simulink model "FloatingOffshoreWind_ForceRAO"  (R2020b)
settings: Solver=ode4  StartTime=0.0  StopTime=200  FixedStep=0.1  RelTol=1e-3  EnableMultiTasking=on
undefined symbols (not defined in the file): slcm, vessel, vesselABC
libraries: simulink_extras x6, mssSimulink x5, simulink x1
settings Model: Creator=Thor  LastModifiedBy=thor
settings DataIOCC: LimitDataPoints=on  SaveFormat=Array  SignalLoggingSaveFormat=ModelDataLogs  ReturnWorkspaceOutputs=off
settings OptimizationCC: ExpressionDepthLimit=2147483647  LifeSpan=inf
settings DebuggingCC: UnderspecifiedInitializationDetection=Classic  MergeDetectMultiDrivingBlocksExec=none  SolverPrmCheckMsg=warning  FcnCallInpInsideContextMsg=warning  StateNameClashWarn=warning  SFUnexpectedBacktrackingDiag=warning  SFNoUnconditionalDefaultTransitionDiag=warning  SFExecutionAtInitializationDiag=none  ArithmeticOperatorsInVariantConditions=warning
settings HardwareCC: ProdBitPerPointer=32  ProdBitPerSizeT=32  ProdBitPerPtrDiffT=32  ProdLargestAtomicFloat=None  ProdIntDivRoundTo=Undefined  ProdEndianess=Unspecified  ProdWordSize=32  ProdHWDeviceType=32-bit Generic
settings ModelReferenceCC: PropagateSignalLabelsOutOfModel=off
settings SFSimCC: SimUseLocalCustomCode=off  CustomCodeUndefinedFunction=UseInterfaceOnly
settings RTWCC: RTWUseLocalCustomCode=off
settings CodeAppCC: StateflowObjectComments=on
settings GRTTargetCC: TargetLangStandard=C89/C90 (ANSI)  CombineOutputUpdateFcns=off  GRTInterface=on
settings ConfigComp: CovMetricSettings=dw  CovSaveCumulativeToWorkspaceVar=on  CovSaveSingleToWorkspaceVar=on

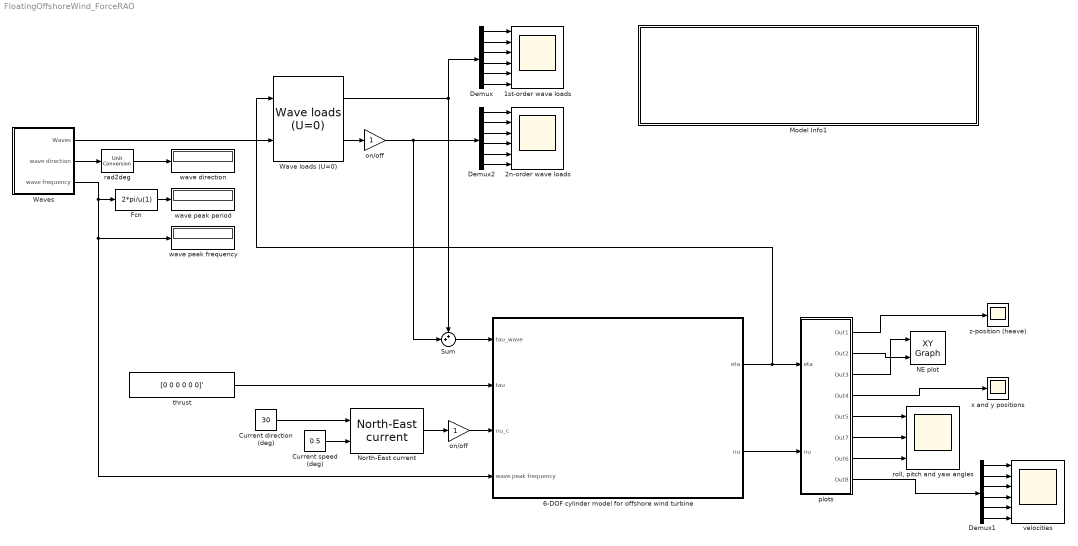
== system FloatingOffshoreWind_ForceRAO ==
  "1st-order wave loads " : Scope  NumInputPorts=6
  2n-order wave loads : Scope  NumInputPorts=6
  6-DOF cylinder model for offshore wind turbine : Subsystem  mask(6 DOF zero speed model){}
      mask help: System block containing the zero speed 6 DOF equations of motion.
      mask init:
      | load cylinder;
      | load cylinderABC;
      | ABC = vesselABC;
      mask Display: image('windturbine.jpg'); % Use "Edit Image" on toolstrip to change.
  Current direction (deg) : Constant  Value=30
  Current speed (deg) : Constant  Value=0.5
  Demux : Demux  Outputs=6
      settings: DisplayOption=none
  Demux1 : Demux  Outputs=6
      settings: DisplayOption=none
  Demux2 : Demux  Outputs=6
      settings: DisplayOption=none
  Fcn : Fcn  Expr=2*pi/u(1)
  Model Info1 : Subsystem  LoadFcn=slcm LoadBlock;  InitFcn=slcm('UpdateAllCMBlocksInThisModelInit')  mask(CMBlock){InitialSaveTempField=, InitialBlockCM=None, BlockCM=None, Frame=on, SaveTempField=, DisplayStringWithTags=|, MaskDisplayString=Offshore wind turbine modelled as a cylinder (D = 10.0 and T = 100.0 m) in WAMIT. \nThe wave-induced motions are computed using force RAOs. \n\nThe vessel simulator for stationkeeping in 6 DOFs is based on frequency-dependent hydrodynamic data. \nThe wave loads are computed using WAMIT data that are postprocessed by:\n\n>> vessel = wamit2vessel ('cylinder',100,10,10) generates the data structure 'vessel'\n\nThe data files are automatically loaded to the workspace before starting the simulation.\n\nAuthor: Thor I. Fossen\nTue Mar 09 08:00:28 2021, HorizontalTextAlignment=Left, LeftAlignmentValue=0.02, SourceBlockDiagram=DP_MotionRAO, TagMaxNumber=20, CMTag1=, CMTag2=, CMTag3=, CMTag4=, CMTag5=, CMTag6=, CMTag7=, CMTag8=, CMTag9=, CMTag10=, CMTag11=, CMTag12=, CMTag13=, CMTag14=, CMTag15=, CMTag16=, CMTag17=, CMTag18=, CMTag19=, CMTag20=}
      mask DisplayStringWithTags=|
      | Offshore wind turbine modelled as a cylinder (D = 10.0 and T = 100.0 m) in WAMIT.
      | The wave-induced motions are computed using force RAOs.
      |
      | The vessel simulator for stationkeeping in 6 DOFs is based on frequency-dependent hydrodynamic data.
      | The wave loads are computed using WAMIT data that are postprocessed by:
      |
      | >> vessel = wamit2vessel ('cylinder',100,10,10) generates the data structure 'vessel'
      |
      | The data files are automatically loaded to the workspace before starting the simulation.
      |
      | Author: Thor I. Fossen
      | %<LastModificationDate>
      mask help: This block allows revision control information to be displayed within the model.
      settings: CopyFcn=slcm CopyBlock;  DeleteFcn=slcm Cancel;  PostSaveFcn=slcm('UpdateAllCMBlocksInThisModel')  NameChangeFcn=slcm Rename;  OpenFcn=slcm
      mask Display: text(str2num(LeftAlignmentValue), 0.5, MaskDisplayString, 'HorizontalAlignment', HorizontalTextAlignment)
  NE plot : simulink/Sinks/XY Graph  xmin=-50  xmax=50  ymin=-50  ymax=50  st=-1
  "North-East current " : mssSimulink/Environment/Current/North-East current  SystemSampleTime=-1  VariantActivationTime=update diagram  Latency=0  AutoFrameSizeCalculation=off
  Sum : Sum  Inputs=++|
  "Wave loads (U=0) " : mssSimulink/Hydrodynamics/Wave loads (U=0)  SystemSampleTime=-1  VariantActivationTime=update diagram  Latency=0  AutoFrameSizeCalculation=off
  Waves : Subsystem  mask(Waves){spectrum_type=Jonswap, disp_flag=off, plot_spectrum=off, plot_realization=off, hs=5, omega_peak=2*pi/8, psi_mean=30*pi/180, gamma=3.3, spread=2, depth=inf, nfreq=20, ndir=10, energylim=0.005, freq_cutoff=3, dir_cutoff=0, rand_seed=0, rand_freq=on, rand_dir=on, Zeta_a=0, Omega=0, Phase=0, Wavenum=0, Psi=0}
      mask prompts: spectrum_type "Spectrum type"; disp_flag "Display initialization info in workspace window"; plot_spectrum "Plot spectrum"; plot_realization "Plot sea state realization (time-consuming)"; hs "Significant wave height Hs (m)"; omega_peak "Peak frequency omega_0 (rad/s)"; psi_mean "Mean wave direction (rad)"; gamma "Spectrum peakedness factor [1,7], 3.3 default, 0 for using DNV value"; spread "Wave spreading factor (1,2,3,4,5)"; depth "Average water depth (m), use inf for deep water"; nfreq "Number of frequencies in grid (recommended > 20)"; ndir "Number of directions in grid, 1 for long-crested waves"; energylim "Wave component energy limit [0 1] or number of waves (e.g. 50)"; freq_cutoff "Frequency cutoff factor [1.5, 5], default 3"; dir_cutoff "Direction cutoff [0, 3pi/8], default 0"; rand_seed "Random seed"; rand_freq "Random frequencies"; rand_dir "Random directions"; Zeta_a "Amplitude vector 'Zeta_a' (m)"; Omega "Frequency vector 'Omega' (rad/s)"; Phase "Phase vector 'Phase' (rad)"; Wavenum "Wavenumber vector 'Wavenum' (1/m)"; Psi "Direction vector 'Psi'  (rad)"
      mask help:
      | Calculate harmonic wave component parameters from a wave spectrum.
      | - Input one wave direction in the mask to get long-crested waves.
      | - Input zero peak frequency to get an expectation value from north sea statistical data.
      | - Input an integer > 1 for energylim to set the number of wave components fixed to nwaves = energylim.
      |
      | Copyright (C) 2004 NTNU
      | Author: Oyvind Notland Smogeli
      mask init:
      | if spectrum_type < 4
      | 	[Zeta_a, Omega, Phase, Wavenum, Psi] = Wave_init(spectrum_type, hs, omega_peak, psi_mean,...
      | 	gamma, spread, depth, nfreq, ndir, energylim, freq_cutoff, dir_cutoff, rand_freq, rand_dir,...
      | 	rand_seed, plot_spectrum, plot_realization, disp_flag);
      | end
      mask Help:
      | <font face="Arial">
      | <b>Project:</b> Marine Systems Simulator: MSS<br>
      | <br>
      | Define harmonic wave components describing the sea state by extracting
      | components from a given frequency and direction spectrum. The output from the
      | block is a bus containing the following wave parameter vectors:</font></p>
      | <p><font face="Arial"><b>Zeta_a</b>: Vector of harmonic wave amplitudes [m]<br>
      | <b>Omega: </b>Vector of harmonic wave frequencies [rad/s]<br>
      | <b>Phase: </b>Vector of harmonic wave phases (random) [rad]<br>
      | <b>Wavenum:</b> Vector of harmonic wave numbers [1/m]<br>
      | <b>Psi: </b>Vector of harmonic wave directions [rad]</font></p>
      | <p><font face="Arial">The time series of sea surface elevation Zeta(x,y,t) can
      | be obtained as</font></p>
      | <p><font face="Arial">Zeta(x,y,t) = Sum( Zeta_a(i)*cos(Omega(i)*t + Phase(i) - Wavenum(i)*(x*cos(Psi(i))
      | + y*sin(Psi(i)))) )</font></p>
      | <p><font face="Arial">where the sum is taken from i = 1 to i = n and n is the number of harmonic
      | wave components.</font></p>
      | <p>&nbsp;</p>
      | <p><font face="Arial">Input one wave direction to get long-crested waves.<br>
      | <br>
      | If the peak frequency is set to zero, then the peak frequency is obtained from
      | the sugnificant wave height usign a formula for the North Sea (Norsok):</font></p>
      | <p><font face="Arial">w0 = 2*pi/(4.883 + 2.68*Hs^0.54);</font></p>
      | 
      | <p>&nbsp;</p>
      | <p><font face="Arial">The energy limit (energylim) should be defined either as a positive factor
      | between 0 and 1, or as a positive integer. In the first case it will
      | discard all wave components with energy content less than this ratio of the
      | total energy content of the sea state. A recommended value is 0.005 or lower. In
      | the second case it will keep the nwaves = energylim most significant waves.</font></p>
      | <p>&nbsp;</p>
      | <p><font face="Arial">The wave elevation Zeta(x,y,t) at time t and at the coordinate (x,y) is found from the output vectors as:</font></p>
      | <p>&nbsp;</p>
      | <p><font face="Arial" color="#800000">References</font><ul>
      |   <li><font face="Arial">Sørensen, A.J. (2005) Lecture notes of TMR4240 &quot;Marine Cybernetics - Modelling and Control&quot;</font>
      |   <font face="Arial">Dept of Marine Technology NTNU.</font></li>
      |   <li><font face="Arial">Johannessen, K., T. S. Meling, S. Haver. Joint
      |   Distribution for Wind and<br>
      |   Waves in the Northern North Sea. IJOPE Vol. 12, No. 1, March 2002</font></li>
      |   <li>&nbsp;</li>
      |   </ul>
      | <p><font face="Arial">Johannessen, K., T. S. Meling, S. Haver. Joint
      | Distribution for Wind and<br>
      | Waves in the Northern North Sea. IJOPE Vol. 12, No. 1, March 2002</font><p>&nbsp;<p>
      |   <font face="Arial"><b>Author:</b> Øyvind Smogeli, September 2004 </font>
      | <p>&nbsp;</p>
      | <p>&nbsp;</p>
      mask TypeOptions spectrum_type: ITTC | Jonswap | Torsethaugen | Predefined waves
      mask Callback spectrum_type: Wave_callback;
  on/off : Gain
  "on/off " : Gain
  plots : Subsystem
      mask Display: disp('time-series')
  rad2deg : mssSimulink/Utilities/Math Operations/Unit Conversion  in=rad2deg
  "roll, pitch and yaw angles" : Scope  NumInputPorts=3
  thrust : Constant  Value=[0 0 0 0 0 0]'
  velocities : Scope  NumInputPorts=6
  wave direction : Display
  wave peak frequency : Display
  wave peak period : Display
  x and y positions : Scope
  z-position (heave) : Scope
  wires:
  plots/3(Out3) -> NE plot/1
  plots/2(Out2) -> NE plot/2
  plots/4(Out4) -> x and y positions/1
  plots/5(Out5) -> "roll, pitch and yaw angles"/1
  plots/6(Out7) -> "roll, pitch and yaw angles"/2
  plots/7(Out6) -> "roll, pitch and yaw angles"/3
  plots/1(Out1) -> z-position (heave)/1
  Demux1/1 -> velocities/1
  Demux1/2 -> velocities/2
  Demux1/3 -> velocities/3
  Demux1/4 -> velocities/4
  Demux1/5 -> velocities/5
  Demux1/6 -> velocities/6
  plots/8(Out8) -> Demux1/1
  6-DOF cylinder model for offshore wind turbine/1(eta) -> "Wave loads (U=0) "/1, plots/1(eta)
  6-DOF cylinder model for offshore wind turbine/2(nu) -> plots/2(nu)
  Demux/1 -> "1st-order wave loads "/1
  Demux/2 -> "1st-order wave loads "/2
  Demux/3 -> "1st-order wave loads "/3
  Demux/4 -> "1st-order wave loads "/4
  Demux/5 -> "1st-order wave loads "/5
  Demux/6 -> "1st-order wave loads "/6
  "Wave loads (U=0) "/2 -> on/off/1
  Waves/1(Waves) -> "Wave loads (U=0) "/2
  Waves/2(wave direction) -> rad2deg/1
  rad2deg/1 -> wave direction/1
  Demux2/1 -> 2n-order wave loads/1
  Demux2/2 -> 2n-order wave loads/2
  Demux2/3 -> 2n-order wave loads/3
  Demux2/4 -> 2n-order wave loads/4
  Demux2/5 -> 2n-order wave loads/5
  Demux2/6 -> 2n-order wave loads/6
  "Wave loads (U=0) "/1 -> Sum/1, Demux/1
  on/off/1 -> Demux2/1, Sum/2
  thrust/1 -> 6-DOF cylinder model for offshore wind turbine/2(tau)
  "North-East current "/1 -> "on/off "/1
  "on/off "/1 -> 6-DOF cylinder model for offshore wind turbine/3(nu_c)
  Current speed (deg)/1 -> "North-East current "/2
  Current direction (deg)/1 -> "North-East current "/1
  Sum/1 -> 6-DOF cylinder model for offshore wind turbine/1(tau_wave)
  Waves/3(wave frequency) -> Fcn/1, 6-DOF cylinder model for offshore wind turbine/4(wave peak frequency), wave peak frequency/1
  Fcn/1 -> wave peak period/1

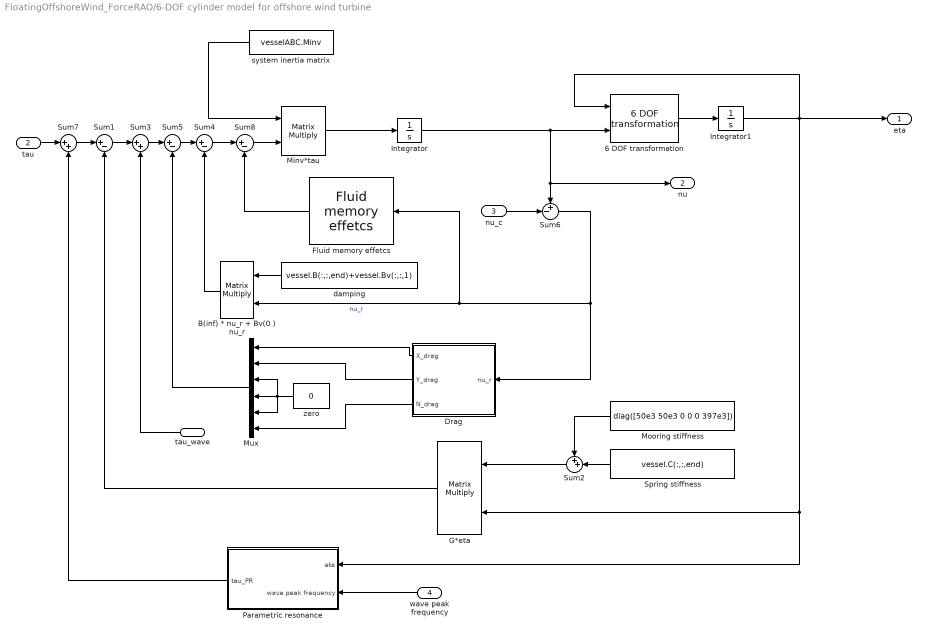
== system FloatingOffshoreWind_ForceRAO/6-DOF cylinder model for offshore wind turbine ==
  tau_wave : Inport
  tau : Inport  Port=2
  nu_c : Inport  Port=3
  wave peak frequency : Inport  Port=4
  "6 DOF transformation " : mssSimulink/Modelling/Kinematics/6 DOF transformation  SystemSampleTime=-1  VariantActivationTime=update diagram  Latency=0  AutoFrameSizeCalculation=off
  "B(inf) * nu_r + Bv(0 ) nu_r " : Product  Multiplication=Matrix(*)  SaturateOnIntegerOverflow=on  OutDataTypeStr=Inherit: Same as first input
  Drag : Subsystem  TreatAsAtomicUnit=on
  Fluid memory effetcs : mssSimulink/Hydrodynamics/Fluid memory effetcs  SystemSampleTime=-1  VariantActivationTime=update diagram  Latency=0  AutoFrameSizeCalculation=off
  G*eta : Product  Multiplication=Matrix(*)  SaturateOnIntegerOverflow=on  OutDataTypeStr=Inherit: Same as first input
  Integrator : Integrator  InitialCondition=[0.001 0.001 0.001 0.001 0.001 0.001]
  Integrator1 : Integrator
  Minv*tau : Product  Inputs=**  Multiplication=Matrix(*)  SaturateOnIntegerOverflow=on  OutDataTypeStr=Inherit: Same as first input
  Mooring stiffness : Constant  Value=diag([50e3 50e3 0 0 0 397e3])
  Mux : Mux  Inputs=6
  Parametric resonance : Subsystem
  Spring stiffness : Constant  Value=vessel.C(:,:,end)
  Sum{1,4..5,8} (4 alike) : Sum  Inputs=|+-  SaturateOnIntegerOverflow=on
  Sum2 : Sum  Inputs=++|  SaturateOnIntegerOverflow=on
  Sum3 : Sum  Inputs=|++  SaturateOnIntegerOverflow=on
  Sum6 : Sum  Inputs=+-|  SaturateOnIntegerOverflow=on
  Sum7 : Sum  Inputs=|++  SaturateOnIntegerOverflow=on
  damping : Constant  Value=vessel.B(:,:,end)+vessel.Bv(:,:,1)
  system inertia matrix : Constant  Value=vesselABC.Minv
  zero : Constant  Value=0
  eta : Outport
  nu : Outport  Port=2
  wires:
  "B(inf) * nu_r + Bv(0 ) nu_r "/1 -> Sum4/2
  Sum3/1 -> Sum5/1
  tau_wave/1 -> Sum3/2
  G*eta/1 -> Sum1/2
  Integrator1/1 -> eta/1, G*eta/2, Parametric resonance/1(eta), "6 DOF transformation "/1
  Spring stiffness/1 -> Sum2/2
  Sum1/1 -> Sum3/1
  Integrator/1 -> nu/1, Sum6/1, "6 DOF transformation "/2
  Drag/1(X_drag) -> Mux/1
  Drag/2(Y_drag) -> Mux/2
  Drag/3(N_drag) -> Mux/6
  zero/1 -> Mux/4, Mux/3, Mux/5
  Mux/1 -> Sum5/2
  Sum5/1 -> Sum4/1
  nu_c/1 -> Sum6/2
  Sum6/1 -> Fluid memory effetcs/1, "B(inf) * nu_r + Bv(0 ) nu_r "/2, Drag/1(nu_r)  "nu_r"
  tau/1 -> Sum7/1
  damping/1 -> "B(inf) * nu_r + Bv(0 ) nu_r "/1
  system inertia matrix/1 -> Minv*tau/1
  Minv*tau/1 -> Integrator/1
  "6 DOF transformation "/1 -> Integrator1/1
  Mooring stiffness/1 -> Sum2/1
  Sum2/1 -> G*eta/1
  Parametric resonance/1(tau_PR) -> Sum7/2
  Sum7/1 -> Sum1/1
  wave peak frequency/1 -> Parametric resonance/2(wave peak frequency)
  Sum4/1 -> Sum8/1
  Sum8/1 -> Minv*tau/2
  Fluid memory effetcs/1 -> Sum8/2

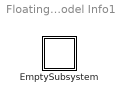
== system FloatingOffshoreWind_ForceRAO/Model Info1 ==
  EmptySubsystem : Subsystem

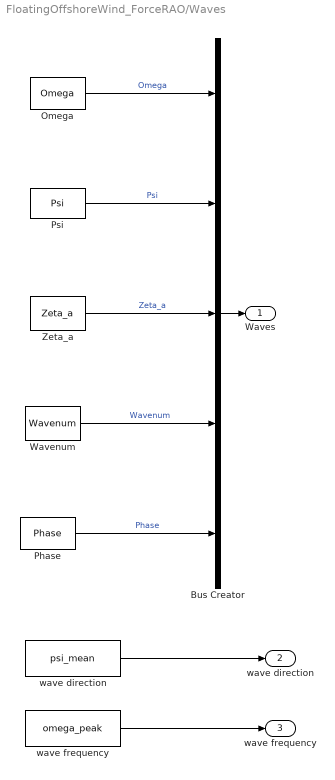
== system FloatingOffshoreWind_ForceRAO/Waves ==
  Bus Creator : BusCreator  Inputs=5
  Omega : Constant  Value=Omega
  Phase : Constant  Value=Phase
  Psi : Constant  Value=Psi
  Wavenum : Constant  Value=Wavenum
  Zeta_a : Constant  Value=Zeta_a
  "wave direction " : Constant  Value=psi_mean
  "wave frequency  " : Constant  Value=omega_peak
  Waves : Outport
  wave direction : Outport  Port=2
  wave frequency : Outport  Port=3
  wires:
  "wave direction "/1 -> wave direction/1
  Wavenum/1 -> Bus Creator/4  "Wavenum"
  Zeta_a/1 -> Bus Creator/3  "Zeta_a"
  Bus Creator/1 -> Waves/1
  Omega/1 -> Bus Creator/1  "Omega"
  Psi/1 -> Bus Creator/2  "Psi"
  Phase/1 -> Bus Creator/5  "Phase"
  "wave frequency  "/1 -> wave frequency/1

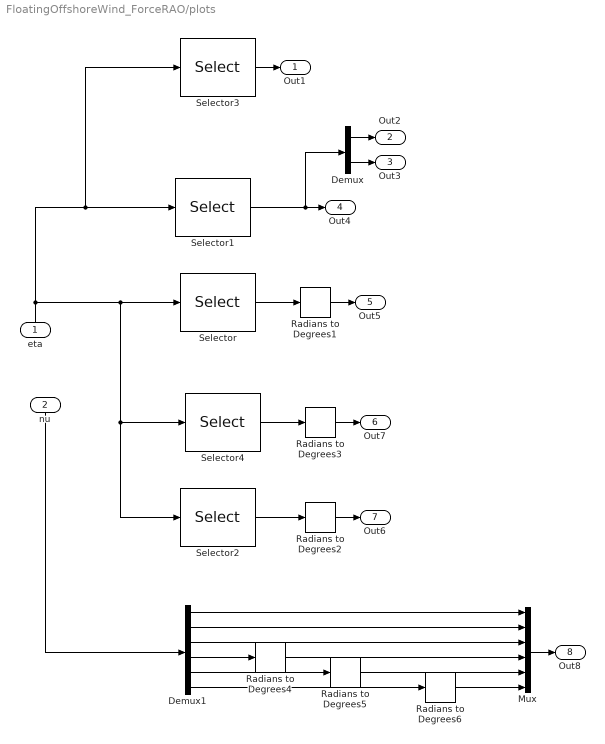
== system FloatingOffshoreWind_ForceRAO/plots ==
  eta : Inport
  nu : Inport  Port=2
  Demux : Demux  Outputs=2
      settings: DisplayOption=none
  Demux1 : Demux  Outputs=6
      settings: DisplayOption=none
  Mux : Mux  Inputs=6
  Radians to Degrees{1..6} (6 alike) : simulink_extras/Transformations/Radians to Degrees
  Selector : Selector  InputPortWidth=6  IndexOptions=Index vector (dialog)  Indices=[4 ]  OutputSizes=1
  Selector1 : Selector  InputPortWidth=6  IndexOptions=Index vector (dialog)  Indices=[1 2]  OutputSizes=1
  Selector2 : Selector  InputPortWidth=6  IndexOptions=Index vector (dialog)  Indices=[6]  OutputSizes=1
  Selector3 : Selector  InputPortWidth=6  IndexOptions=Index vector (dialog)  Indices=[3]  OutputSizes=1
  Selector4 : Selector  InputPortWidth=6  IndexOptions=Index vector (dialog)  Indices=[5]  OutputSizes=1
  Out1 : Outport
  Out2 : Outport  Port=2
  Out3 : Outport  Port=3
  Out4 : Outport  Port=4
  Out5 : Outport  Port=5
  Out7 : Outport  Port=6
  Out6 : Outport  Port=7
  Out8 : Outport  Port=8
  wires:
  eta/1 -> Selector3/1, Selector1/1, Selector/1, Selector2/1, Selector4/1
  Selector/1 -> Radians to Degrees1/1
  Selector1/1 -> Demux/1, Out4/1
  Selector2/1 -> Radians to Degrees2/1
  Selector3/1 -> Out1/1
  Demux/1 -> Out2/1
  Demux/2 -> Out3/1
  Radians to Degrees1/1 -> Out5/1
  Radians to Degrees2/1 -> Out6/1
  Selector4/1 -> Radians to Degrees3/1
  Radians to Degrees3/1 -> Out7/1
  nu/1 -> Demux1/1
  Demux1/1 -> Mux/1
  Demux1/2 -> Mux/2
  Demux1/3 -> Mux/3
  Demux1/4 -> Radians to Degrees4/1
  Demux1/5 -> Radians to Degrees5/1
  Demux1/6 -> Radians to Degrees6/1
  Radians to Degrees6/1 -> Mux/6
  Radians to Degrees5/1 -> Mux/5
  Radians to Degrees4/1 -> Mux/4
  Mux/1 -> Out8/1

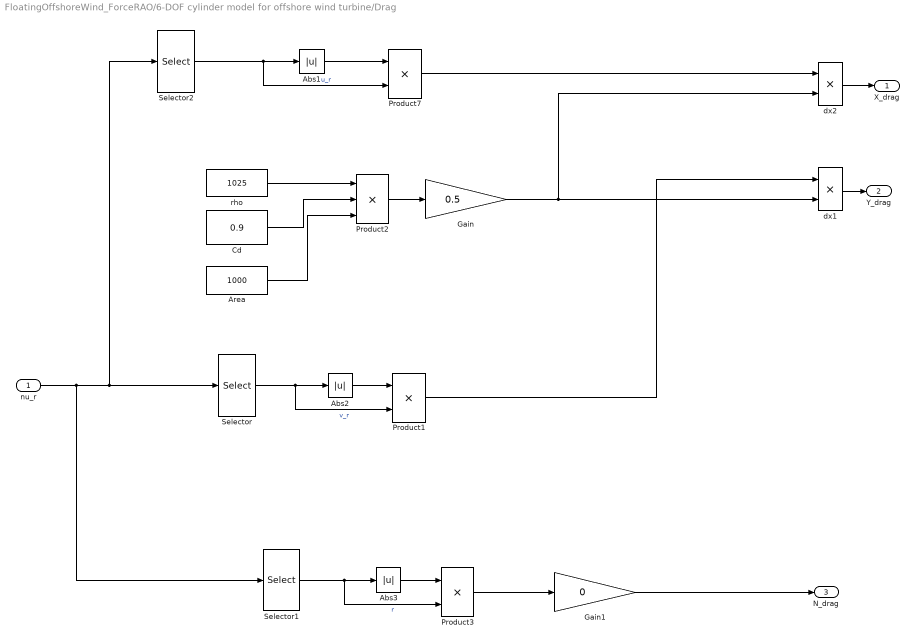
== system FloatingOffshoreWind_ForceRAO/6-DOF cylinder model for offshore wind turbine/Drag ==
  nu_r : Inport
  Abs1 : Abs  SaturateOnIntegerOverflow=on
  Abs2 : Abs  SaturateOnIntegerOverflow=on
  Abs3 : Abs  SaturateOnIntegerOverflow=on
  Area : Constant  Value=1000
  Cd : Constant  Value=0.9
  Gain : Gain  Gain=0.5  SaturateOnIntegerOverflow=on  OutDataTypeStr=Inherit: Same as input  ParamDataTypeStr=Inherit: Same as input
  Gain1 : Gain  Gain=0  SaturateOnIntegerOverflow=on  OutDataTypeStr=Inherit: Same as input  ParamDataTypeStr=Inherit: Same as input
  Product1 : Product  SaturateOnIntegerOverflow=on  OutDataTypeStr=Inherit: Same as first input
  Product2 : Product  Inputs=3  SaturateOnIntegerOverflow=on  OutDataTypeStr=Inherit: Same as first input
  Product3 : Product  SaturateOnIntegerOverflow=on  OutDataTypeStr=Inherit: Same as first input
  Product7 : Product  SaturateOnIntegerOverflow=on  OutDataTypeStr=Inherit: Same as first input
  Selector : Selector  InputPortWidth=6  IndexOptions=Index vector (dialog)  Indices=[2]  OutputSizes=1
  Selector1 : Selector  InputPortWidth=6  IndexOptions=Index vector (dialog)  Indices=[6]  OutputSizes=1
  Selector2 : Selector  InputPortWidth=6  IndexOptions=Index vector (dialog)  Indices=[1]  OutputSizes=1
  dx1 : Product  RndMeth=Zero
  dx2 : Product  RndMeth=Zero
  rho : Constant  Value=1025
  X_drag : Outport
  Y_drag : Outport  Port=2
  N_drag : Outport  Port=3
  wires:
  dx1/1 -> Y_drag/1
  nu_r/1 -> Selector2/1, Selector/1, Selector1/1
  Selector2/1 -> Product7/2, Abs1/1  "u_r"
  Abs1/1 -> Product7/1
  Selector/1 -> Product1/2, Abs2/1  "v_r"
  Abs2/1 -> Product1/1
  rho/1 -> Product2/1
  Cd/1 -> Product2/2
  Area/1 -> Product2/3
  Product2/1 -> Gain/1
  Gain/1 -> dx1/2, dx2/2
  Product7/1 -> dx2/1
  dx2/1 -> X_drag/1
  Product1/1 -> dx1/1
  Selector1/1 -> Product3/2, Abs3/1  "r"
  Abs3/1 -> Product3/1
  Product3/1 -> Gain1/1
  Gain1/1 -> N_drag/1

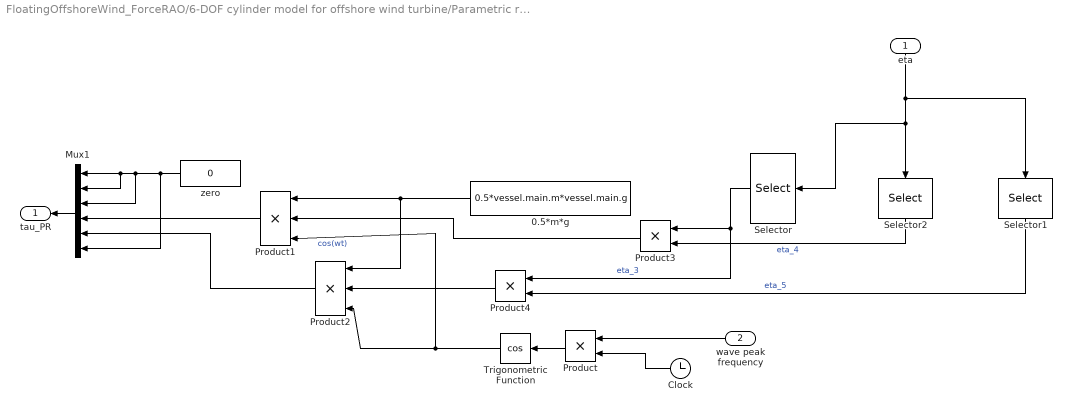
== system FloatingOffshoreWind_ForceRAO/6-DOF cylinder model for offshore wind turbine/Parametric resonance ==
  eta : Inport
  wave peak frequency : Inport  Port=2
  0.5*m*g : Constant  Value=0.5*vessel.main.m*vessel.main.g
  Clock : Clock
  Mux1 : Mux  Inputs=6
  Product : Product  RndMeth=Zero
  Product1 : Product  Inputs=3  RndMeth=Zero
  Product2 : Product  Inputs=3  RndMeth=Zero
  Product3 : Product  RndMeth=Zero
  Product4 : Product  RndMeth=Zero
  Selector : Selector  InputPortWidth=6  IndexOptions=Index vector (dialog)  Indices=[3]  OutputSizes=1
  Selector1 : Selector  InputPortWidth=6  IndexOptions=Index vector (dialog)  Indices=[5]  OutputSizes=1
  Selector2 : Selector  InputPortWidth=6  IndexOptions=Index vector (dialog)  Indices=[4]  OutputSizes=1
  Trigonometric Function : Trigonometry  Operator=cos
  "zero  " : Constant  Value=0
  tau_PR : Outport
  wires:
  0.5*m*g/1 -> Product2/1, Product1/1
  wave peak frequency/1 -> Product/1
  Clock/1 -> Product/2
  Product/1 -> Trigonometric Function/1
  "zero  "/1 -> Mux1/1, Mux1/2, Mux1/3, Mux1/6
  Product1/1 -> Mux1/4
  Trigonometric Function/1 -> Product1/3, Product2/3  "cos(wt)"
  Product2/1 -> Mux1/5
  Selector/1 -> Product3/1, Product4/1  "eta_3"
  Selector2/1 -> Product3/2  "eta_4"
  Selector1/1 -> Product4/2  "eta_5"
  Product3/1 -> Product1/2
  Product4/1 -> Product2/2
  Mux1/1 -> tau_PR/1
  eta/1 -> Selector1/1, Selector2/1, Selector/1

== system FloatingOffshoreWind_ForceRAO/Model Info1/EmptySubsystem ==
